simulink model "model"  (R2024a)
settings: Solver=ode4  StartTime=0.0  StopTime=10.0  RelTol=1e-3
values from neighbouring files (symbols this model uses):
  g = 9.81    [script.m]    (also in srcipt.m)
  h = 0.25    [script.m]    (also in srcipt.m)
  L = 2.6    [script.m]    (also in srcipt.m)
  lf = 2.1    [script.m]    (also in srcipt.m)
  lr = 0.5    [script.m]    (also in srcipt.m)
  ls = 1.242    [script.m]    (also in srcipt.m)
  m = 180    [script.m]    (also in srcipt.m)
  rw = 0.217    [script.m]    (also in srcipt.m)
settings Model: Creator=DELL  LastModifiedBy=DELL
settings OptimizationCC: BlockReduction=off  ConditionallyExecuteInputs=off  StrengthReduction=on  PassReuseOutputArgsAs=Individual arguments  RollThreshold=0  ZeroExternalMemoryAtStartup=off  ZeroInternalMemoryAtStartup=off  OptimizeBlockOrder=speed  OptimizationPriority=Speed  OptimizationCustomize=off  MultiThreadedLoops=on  AutoScheduleForLoops=on  EfficientTunableParamExpr=on
settings DebuggingCC: ParameterTunabilityLossMsg=error
settings SFSimCC: MATLABDynamicMemAlloc=off
settings RTWCC: Description=Embedded Coder  SystemTargetFile=ert.tlc  GenCodeOnly=on  TemplateMakefile=ert_default_tmf
settings CodeAppCC: ForceParamTrailComments=on  IgnoreCustomStorageClasses=off  OperatorAnnotations=on  SimulinkDataObjDesc=on  SFDataObjDesc=on  InsertBlockDesc=on
settings ERTTargetCC: TargetLangStandard=C99 (ISO)  GenerateSampleERTMain=on  SupportContinuousTime=on  ERTCustomFileTemplate=example_file_process.tlc

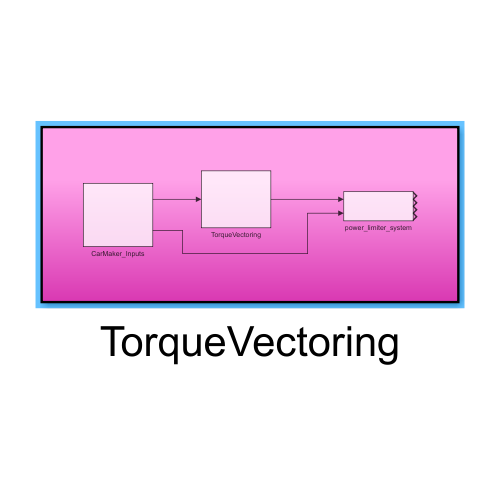
[thumbnail: Simulink's stored preview of the top-level diagram]
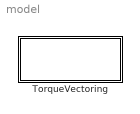
== system model ==
  TorqueVectoring : Subsystem

== system model/TorqueVectoring ==
  CarMaker_Inputs : Subsystem
  TorqueVectoring : Subsystem
  power_limiter_system : Subsystem
  wires:
  CarMaker_Inputs/1(Inputs) -> TorqueVectoring/1(Inputs)
  TorqueVectoring/1(Torques) -> power_limiter_system/1(torques)
  CarMaker_Inputs/2(whls_spd) -> power_limiter_system/2(whls_spd)

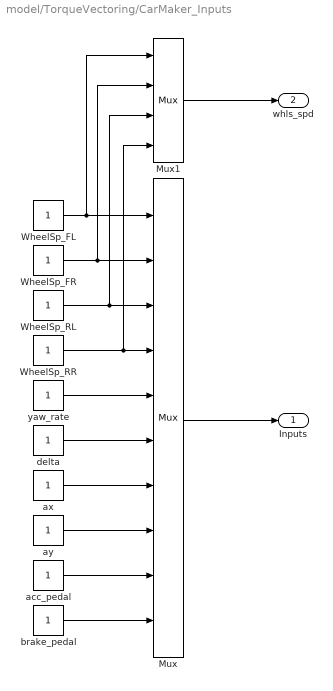
== system model/TorqueVectoring/CarMaker_Inputs ==
  Mux : Mux  Inputs=10
  Mux1 : Mux
  WheelSp_FL : Constant
  WheelSp_FR : Constant
  WheelSp_RL : Constant
  WheelSp_RR : Constant
  acc_pedal : Constant
  ax : Constant
  ay : Constant
  brake_pedal : Constant
  delta : Constant
  yaw_rate : Constant
  Inputs : Outport
  whls_spd : Outport  Port=2
  wires:
  Mux/1 -> Inputs/1
  WheelSp_FL/1 -> Mux1/1, Mux/1
  WheelSp_FR/1 -> Mux1/2, Mux/2
  WheelSp_RL/1 -> Mux1/3, Mux/3
  WheelSp_RR/1 -> Mux1/4, Mux/4
  brake_pedal/1 -> Mux/10
  acc_pedal/1 -> Mux/9
  ax/1 -> Mux/7
  delta/1 -> Mux/6
  yaw_rate/1 -> Mux/5
  ay/1 -> Mux/8
  Mux1/1 -> whls_spd/1

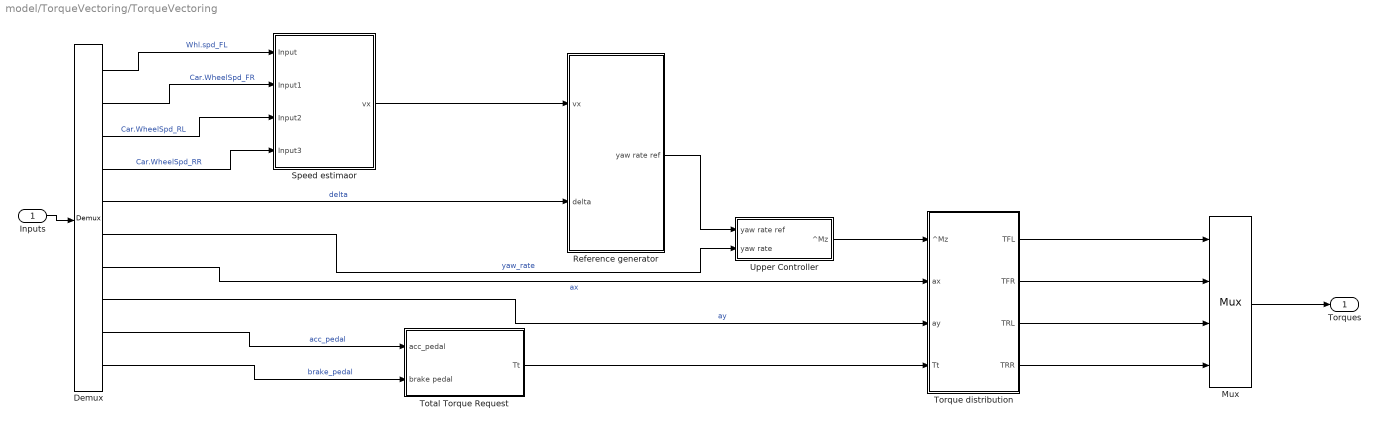
== system model/TorqueVectoring/TorqueVectoring ==
  Inputs : Inport
  Demux : Demux  Outputs=10
  Mux : Mux
  Reference generator : Subsystem
  Speed estimaor : Subsystem
  Torque distribution : Subsystem
  Total Torque Request : Subsystem
  Upper Controller : Subsystem
  Torques : Outport
  wires:
  Reference generator/1(yaw rate ref) -> Upper Controller/1(yaw rate ref)
  Upper Controller/1(^Mz) -> Torque distribution/1(^Mz)
  Total Torque Request/1(Tt) -> Torque distribution/4(Tt)
  Torque distribution/2(TFR) -> Mux/2
  Torque distribution/3(TRL) -> Mux/3
  Torque distribution/4(TRR) -> Mux/4
  Mux/1 -> Torques/1
  Inputs/1 -> Demux/1
  Speed estimaor/1(vx) -> Reference generator/1(vx)
  Demux/1 -> Speed estimaor/1(Input)  "Whl.spd_FL"
  Demux/2 -> Speed estimaor/2(Input1)  "Car.WheelSpd_FR"
  Demux/3 -> Speed estimaor/3(Input2)  "Car.WheelSpd_RL"
  Demux/4 -> Speed estimaor/4(Input3)  "Car.WheelSpd_RR"
  Torque distribution/1(TFL) -> Mux/1
  Demux/5 -> Reference generator/2(delta)  "delta"
  Demux/6 -> Upper Controller/2(yaw rate)  "yaw_rate"
  Demux/7 -> Torque distribution/2(ax)  "ax"
  Demux/8 -> Torque distribution/3(ay)  "ay"
  Demux/9 -> Total Torque Request/1(acc_pedal)  "acc_pedal"
  Demux/10 -> Total Torque Request/2(brake pedal)  "brake_pedal"

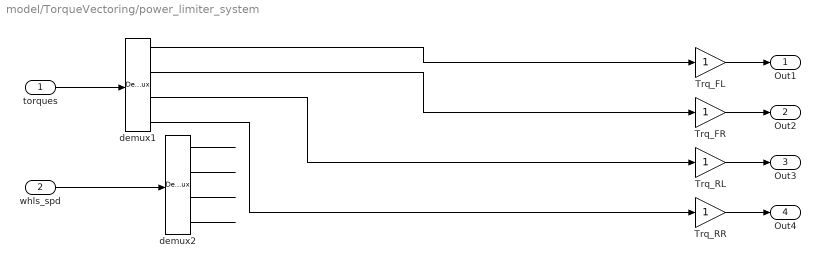
== system model/TorqueVectoring/power_limiter_system ==
  torques : Inport
  whls_spd : Inport  Port=2
  Trq_FL : Gain
  Trq_FR : Gain
  Trq_RL : Gain
  Trq_RR : Gain
  demux1 : Demux
  demux2 : Demux
  Out1 : Outport
  Out2 : Outport  Port=2
  Out3 : Outport  Port=3
  Out4 : Outport  Port=4
  wires:
  demux2/4 -> ?
  demux2/3 -> ?
  demux2/2 -> ?
  demux2/1 -> ?
  torques/1 -> demux1/1
  whls_spd/1 -> demux2/1
  demux1/1 -> Trq_FL/1
  demux1/2 -> Trq_FR/1
  demux1/3 -> Trq_RL/1
  demux1/4 -> Trq_RR/1
  Trq_FL/1 -> Out1/1
  Trq_FR/1 -> Out2/1
  Trq_RR/1 -> Out4/1
  Trq_RL/1 -> Out3/1

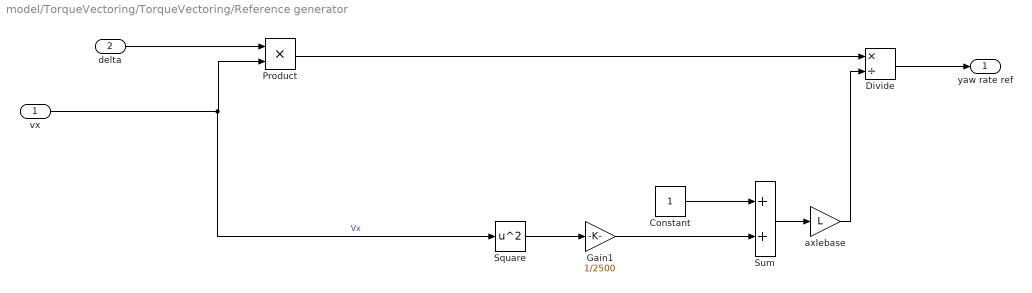
== system model/TorqueVectoring/TorqueVectoring/Reference generator ==
  vx : Inport
  delta : Inport  Port=2
  Constant : Constant
  Divide : Product  Inputs=*/
  Gain1 : Gain  Gain=1/2500
  Product : Product
  Square : Math  Operator=square
  Sum : Sum
  axlebase : Gain  Gain=L
  yaw rate ref : Outport
  wires:
  delta/1 -> Product/1
  Product/1 -> Divide/1
  Constant/1 -> Sum/1
  vx/1 -> Square/1, Product/2  "Vx"
  Square/1 -> Gain1/1
  Gain1/1 -> Sum/2
  Divide/1 -> yaw rate ref/1
  axlebase/1 -> Divide/2
  Sum/1 -> axlebase/1

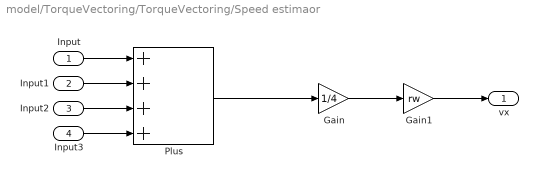
== system model/TorqueVectoring/TorqueVectoring/Speed estimaor ==
  Input : Inport
  Input1 : Inport  Port=2
  Input2 : Inport  Port=3
  Input3 : Inport  Port=4
  Gain : Gain  Gain=1/4
  Gain1 : Gain  Gain=rw
  Plus : Sum  Inputs=++++
  vx : Outport
  wires:
  Input/1 -> Plus/1
  Input1/1 -> Plus/2
  Input3/1 -> Plus/4
  Input2/1 -> Plus/3
  Plus/1 -> Gain/1
  Gain/1 -> Gain1/1
  Gain1/1 -> vx/1

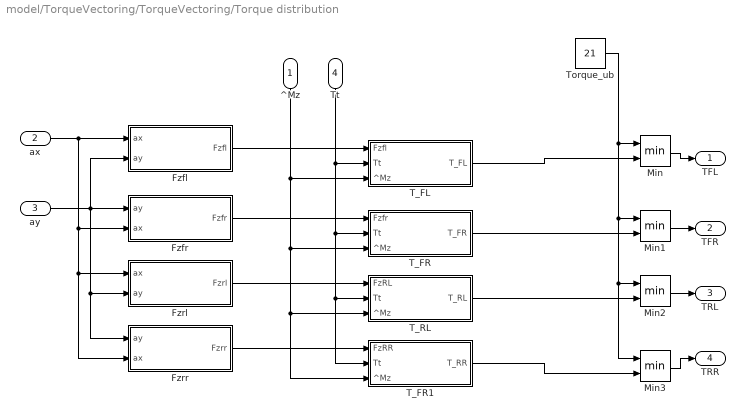
== system model/TorqueVectoring/TorqueVectoring/Torque distribution ==
  ^Mz : Inport
  ax : Inport  Port=2
  ay : Inport  Port=3
  Tt : Inport  Port=4
  Fzfl : Subsystem
  Fzfr : Subsystem
  Fzrl : Subsystem
  Fzrr : Subsystem
  Min{,1..3} (4 alike) : MinMax  Inputs=2
  T_FL : Subsystem
  T_FR : Subsystem
  T_FR1 : Subsystem
  T_RL : Subsystem
  Torque_ub : Constant  Value=21
  TFL : Outport
  TFR : Outport  Port=2
  TRL : Outport  Port=3
  TRR : Outport  Port=4
  wires:
  ax/1 -> Fzrr/2(ax), Fzrl/1(ax), Fzfr/2(ax), Fzfl/1(ax)
  ay/1 -> Fzfl/2(ay), Fzrr/1(ay), Fzrl/2(ay), Fzfr/1(ay)
  Tt/1 -> T_FR1/2(Tt), T_RL/2(Tt), T_FR/2(Tt), T_FL/2(Tt)
  ^Mz/1 -> T_FR1/3(^Mz), T_RL/3(^Mz), T_FR/3(^Mz), T_FL/3(^Mz)
  Fzfl/1(Fzfl) -> T_FL/1(Fzfl)
  Fzfr/1(Fzfr) -> T_FR/1(Fzfr)
  Fzrl/1(Fzrl) -> T_RL/1(FzRL)
  Fzrr/1(Fzrr) -> T_FR1/1(FzRR)
  Torque_ub/1 -> Min3/1, Min2/1, Min1/1, Min/1
  T_FL/1(T_FL) -> Min/2
  Min/1 -> TFL/1
  T_FR1/1(T_RR) -> Min3/2
  Min3/1 -> TRR/1
  Min2/1 -> TRL/1
  T_RL/1(T_RL) -> Min2/2
  Min1/1 -> TFR/1
  T_FR/1(T_FR) -> Min1/2

== system model/TorqueVectoring/TorqueVectoring/Total Torque Request ==
  acc_pedal : Inport
  brake pedal : Inport  Port=2
  Constant1 : Constant  Value=84
  Product1 : Product
  Sum1 : Sum  Inputs=+-
  Tt : Outport
  wires:
  Sum1/1 -> Product1/2
  Product1/1 -> Tt/1
  acc_pedal/1 -> Sum1/1
  Constant1/1 -> Product1/1
  brake pedal/1 -> Sum1/2

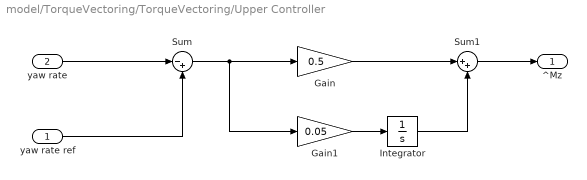
== system model/TorqueVectoring/TorqueVectoring/Upper Controller ==
  yaw rate ref : Inport
  yaw rate : Inport  Port=2
  Gain : Gain  Gain=0.5
  Gain1 : Gain  Gain=0.05
  Integrator : Integrator
  Sum : Sum  Inputs=|-+
  Sum1 : Sum  Inputs=|++
  ^Mz : Outport
  wires:
  yaw rate ref/1 -> Sum/2
  yaw rate/1 -> Sum/1
  Gain1/1 -> Integrator/1
  Integrator/1 -> Sum1/2
  Gain/1 -> Sum1/1
  Sum/1 -> Gain1/1, Gain/1
  Sum1/1 -> ^Mz/1

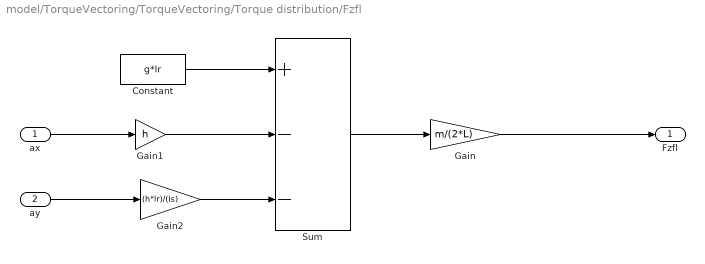
== system model/TorqueVectoring/TorqueVectoring/Torque distribution/Fzfl ==
  ax : Inport
  ay : Inport  Port=2
  Constant : Constant  Value=g*lr
  Gain : Gain  Gain=m/(2*L)
  Gain1 : Gain  Gain=h
  Gain2 : Gain  Gain=(h*lr)/(ls)
  Sum : Sum  Inputs=+--
  Fzfl : Outport
  wires:
  Sum/1 -> Gain/1
  Constant/1 -> Sum/1
  Gain1/1 -> Sum/2
  ax/1 -> Gain1/1
  ay/1 -> Gain2/1
  Gain2/1 -> Sum/3
  Gain/1 -> Fzfl/1

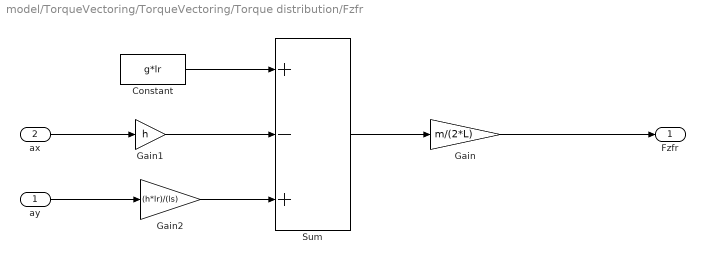
== system model/TorqueVectoring/TorqueVectoring/Torque distribution/Fzfr ==
  ay : Inport
  ax : Inport  Port=2
  Constant : Constant  Value=g*lr
  Gain : Gain  Gain=m/(2*L)
  Gain1 : Gain  Gain=h
  Gain2 : Gain  Gain=(h*lr)/(ls)
  Sum : Sum  Inputs=+-+
  Fzfr : Outport
  wires:
  Sum/1 -> Gain/1
  Constant/1 -> Sum/1
  Gain1/1 -> Sum/2
  ax/1 -> Gain1/1
  ay/1 -> Gain2/1
  Gain2/1 -> Sum/3
  Gain/1 -> Fzfr/1

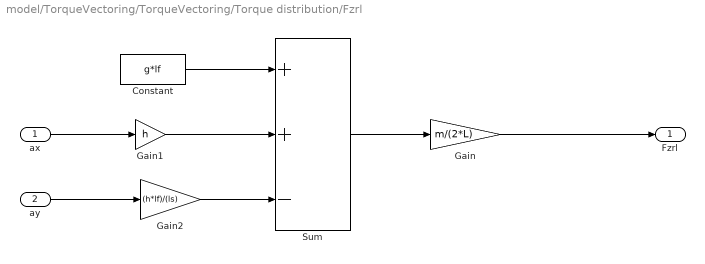
== system model/TorqueVectoring/TorqueVectoring/Torque distribution/Fzrl ==
  ax : Inport
  ay : Inport  Port=2
  Constant : Constant  Value=g*lf
  Gain : Gain  Gain=m/(2*L)
  Gain1 : Gain  Gain=h
  Gain2 : Gain  Gain=(h*lf)/(ls)
  Sum : Sum  Inputs=++-
  Fzrl : Outport
  wires:
  Gain/1 -> Fzrl/1
  Gain2/1 -> Sum/3
  ay/1 -> Gain2/1
  Sum/1 -> Gain/1
  Constant/1 -> Sum/1
  ax/1 -> Gain1/1
  Gain1/1 -> Sum/2

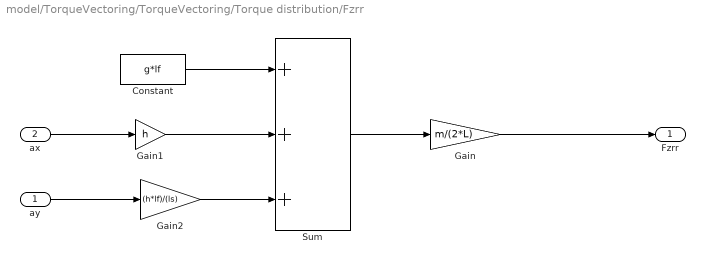
== system model/TorqueVectoring/TorqueVectoring/Torque distribution/Fzrr ==
  ay : Inport
  ax : Inport  Port=2
  Constant : Constant  Value=g*lf
  Gain : Gain  Gain=m/(2*L)
  Gain1 : Gain  Gain=h
  Gain2 : Gain  Gain=(h*lf)/(ls)
  Sum : Sum  Inputs=+++
  Fzrr : Outport
  wires:
  Gain/1 -> Fzrr/1
  Gain2/1 -> Sum/3
  ay/1 -> Gain2/1
  Sum/1 -> Gain/1
  Constant/1 -> Sum/1
  ax/1 -> Gain1/1
  Gain1/1 -> Sum/2

== system model/TorqueVectoring/TorqueVectoring/Torque distribution/T_FL ==
  Fzfl : Inport
  Tt : Inport  Port=2
  ^Mz : Inport  Port=3
  Gain : Gain  Gain=rw/ls
  Gain1 : Gain  Gain=1/(m*g)
  Product : Product
  Sum : Sum  Inputs=+-
  T_FL : Outport
  wires:
  Gain/1 -> Sum/2
  Tt/1 -> Sum/1
  ^Mz/1 -> Gain/1
  Fzfl/1 -> Gain1/1
  Gain1/1 -> Product/1
  Product/1 -> T_FL/1
  Sum/1 -> Product/2

== system model/TorqueVectoring/TorqueVectoring/Torque distribution/T_FR ==
  Fzfr : Inport
  Tt : Inport  Port=2
  ^Mz : Inport  Port=3
  Gain : Gain  Gain=rw/ls
  Gain1 : Gain  Gain=1/(m*g)
  Product : Product
  Sum : Sum
  T_FR : Outport
  wires:
  Gain/1 -> Sum/2
  Tt/1 -> Sum/1
  ^Mz/1 -> Gain/1
  Fzfr/1 -> Gain1/1
  Gain1/1 -> Product/1
  Product/1 -> T_FR/1
  Sum/1 -> Product/2

== system model/TorqueVectoring/TorqueVectoring/Torque distribution/T_FR1 ==
  FzRR : Inport
  Tt : Inport  Port=2
  ^Mz : Inport  Port=3
  Gain : Gain  Gain=rw/ls
  Gain1 : Gain  Gain=1/(m*g)
  Product : Product
  Sum : Sum
  T_RR : Outport
  wires:
  Gain/1 -> Sum/2
  Tt/1 -> Sum/1
  ^Mz/1 -> Gain/1
  FzRR/1 -> Gain1/1
  Gain1/1 -> Product/1
  Product/1 -> T_RR/1
  Sum/1 -> Product/2

== system model/TorqueVectoring/TorqueVectoring/Torque distribution/T_RL ==
  FzRL : Inport
  Tt : Inport  Port=2
  ^Mz : Inport  Port=3
  Gain : Gain  Gain=rw/ls
  Gain1 : Gain  Gain=1/(m*g)
  Product : Product
  Sum : Sum  Inputs=+-
  T_RL : Outport
  wires:
  Gain/1 -> Sum/2
  Tt/1 -> Sum/1
  ^Mz/1 -> Gain/1
  FzRL/1 -> Gain1/1
  Gain1/1 -> Product/1
  Product/1 -> T_RL/1
  Sum/1 -> Product/2
